simulink model "ANNpidSimulation"  (R2024b)
settings: Solver=ode45  StartTime=0.0  StopTime=5  FixedStep=1E-4  MaxStep=1E-4  RelTol=1E-3
undefined symbols (not defined in the file): initial_1, x, y, z
settings Model: Creator=b_ant  LastModifiedBy=b_ant
settings SolverCC: ZeroCrossAlgorithm=Adaptive
settings DebuggingCC: IgnoredZcDiagnostic=none  UnconnectedInputMsg=warning  UnconnectedOutputMsg=warning  UnconnectedLineMsg=warning
settings ModelReferenceCC: EnableRefExpFcnMdlSchedulingChecks=on
settings RTWCC: GPUComputeCapability=3.5  DLArmComputeVersion=19.05

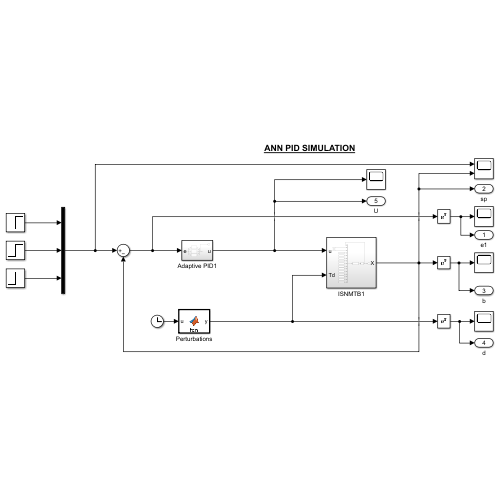
[thumbnail: Simulink's stored preview of the top-level diagram]
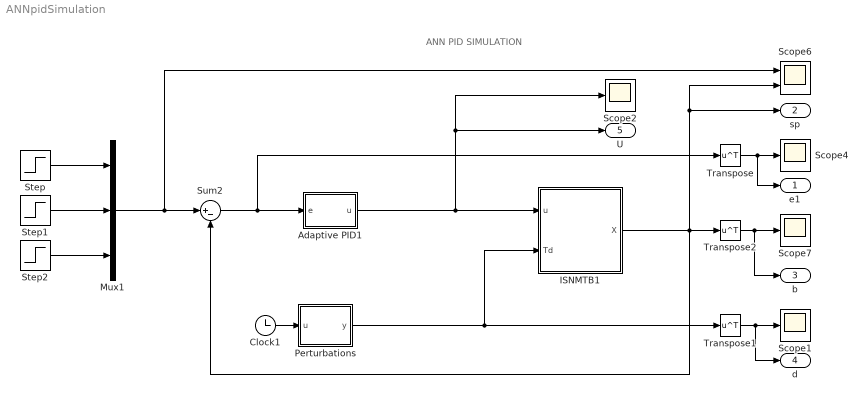
== system ANNpidSimulation ==
  note: ANN PID SIMULATION
  Adaptive PID1 : Subsystem
  Clock1 : Clock
      settings: Decimation=1000
  ISNMTB1 : Subsystem
  Mux1 : Mux  Inputs=3
  Perturbations : MATLAB Function  TreatAsAtomicUnit=on
  Scope{1..2,4,7} (4 alike) : Scope
  Scope6 : Scope  NumInputPorts=2
  Step : Step  Time=0.1  SampleTime=0
  Step1 : Step  Time=0.1  SampleTime=0
  Step2 : Step  Time=0.1  SampleTime=0
  Sum2 : Sum  Inputs=|+-
  Transpose : Math  Operator=transpose
  Transpose1 : Math  Operator=transpose
  Transpose2 : Math  Operator=transpose
  e1 : Outport
  sp : Outport  Port=2
  b : Outport  Port=3
  d : Outport  Port=4
  U : Outport  Port=5
  wires:
  Transpose1/1 -> Scope1/1, d/1
  ISNMTB1/1(X) -> sp/1, Scope6/2, Sum2/2, Transpose2/1
  Sum2/1 -> Transpose/1, Adaptive PID1/1(e)
  Step2/1 -> Mux1/3
  Transpose2/1 -> Scope7/1, b/1
  Step1/1 -> Mux1/2
  Clock1/1 -> Perturbations/1(u)
  Transpose/1 -> e1/1, Scope4/1
  Step/1 -> Mux1/1
  Mux1/1 -> Sum2/1, Scope6/1
  Perturbations/1(y) -> ISNMTB1/2(Td), Transpose1/1
  Adaptive PID1/1(u) -> U/1, Scope2/1, ISNMTB1/1(u)

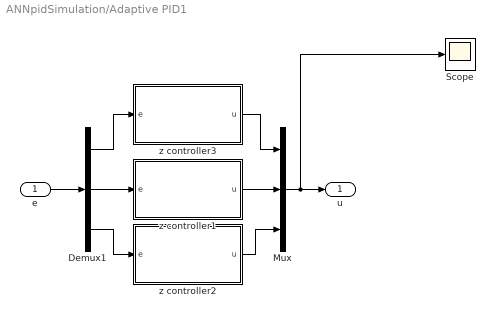
== system ANNpidSimulation/Adaptive PID1 ==
  e : Inport
  Demux1 : Demux  Outputs=3
  Mux : Mux  Inputs=3
  Scope : Scope
  z controller1 : Subsystem
  z controller2 : Subsystem
  z controller3 : Subsystem
  u : Outport
  wires:
  Demux1/2 -> z controller1/1(e)
  z controller3/1(u) -> Mux/1
  e/1 -> Demux1/1
  Demux1/1 -> z controller3/1(e)
  Mux/1 -> Scope/1, u/1
  Demux1/3 -> z controller2/1(e)
  z controller1/1(u) -> Mux/2
  z controller2/1(u) -> Mux/3

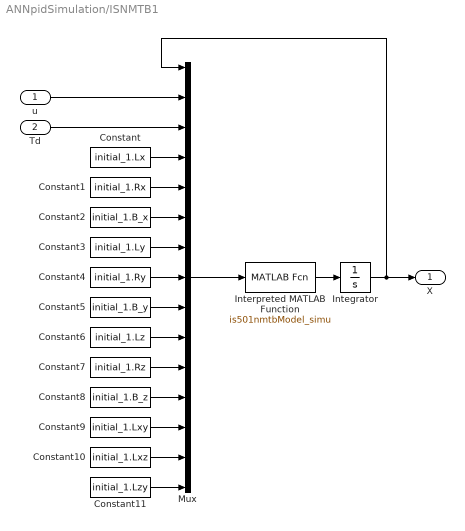
== system ANNpidSimulation/ISNMTB1 ==
  u : Inport
  Td : Inport  Port=2
  Constant : Constant  Value=initial_1.Lx
  Constant1 : Constant  Value=initial_1.Rx
  Constant10 : Constant  Value=initial_1.Lxz
  Constant11 : Constant  Value=initial_1.Lzy
  Constant2 : Constant  Value=initial_1.B_x
  Constant3 : Constant  Value=initial_1.Ly
  Constant4 : Constant  Value=initial_1.Ry
  Constant5 : Constant  Value=initial_1.B_y
  Constant6 : Constant  Value=initial_1.Lz
  Constant7 : Constant  Value=initial_1.Rz
  Constant8 : Constant  Value=initial_1.B_z
  Constant9 : Constant  Value=initial_1.Lxy
  Integrator : Integrator  InitialCondition=[3.249E4, -2.265E4, 3.655E4]
  Interpreted MATLAB Function : MATLABFcn  MATLABFcn=is501nmtbModel_simu
  Mux : Mux  Inputs=15
  X : Outport
  wires:
  Interpreted MATLAB Function/1 -> Integrator/1
  Integrator/1 -> X/1, Mux/1
  Mux/1 -> Interpreted MATLAB Function/1
  u/1 -> Mux/2
  Td/1 -> Mux/3
  Constant/1 -> Mux/4
  Constant1/1 -> Mux/5
  Constant2/1 -> Mux/6
  Constant3/1 -> Mux/7
  Constant4/1 -> Mux/8
  Constant5/1 -> Mux/9
  Constant6/1 -> Mux/10
  Constant7/1 -> Mux/11
  Constant8/1 -> Mux/12
  Constant9/1 -> Mux/13
  Constant10/1 -> Mux/14
  Constant11/1 -> Mux/15

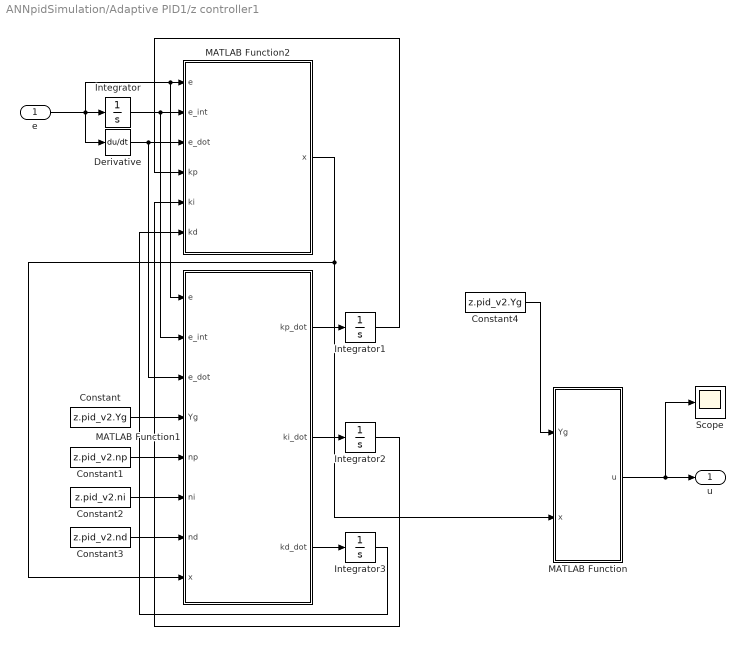
== system ANNpidSimulation/Adaptive PID1/z controller1 ==
  e : Inport
  Constant : Constant  Value=z.pid_v2.Yg
  Constant1 : Constant  Value=z.pid_v2.np
  Constant2 : Constant  Value=z.pid_v2.ni
  Constant3 : Constant  Value=z.pid_v2.nd
  Constant4 : Constant  Value=z.pid_v2.Yg
  Derivative : Derivative
  Integrator : Integrator
  Integrator1 : Integrator  InitialCondition=y.PID.Kp
  Integrator2 : Integrator  InitialCondition=y.PID.Ki
  Integrator3 : Integrator  InitialCondition=y.PID.Kd
  MATLAB Function : MATLAB Function  TreatAsAtomicUnit=on
  MATLAB Function1 : MATLAB Function  TreatAsAtomicUnit=on
  MATLAB Function2 : MATLAB Function  TreatAsAtomicUnit=on
  Scope : Scope
  u : Outport
  wires:
  e/1 -> Derivative/1, Integrator/1, MATLAB Function1/1(e), MATLAB Function2/1(e)
  Constant/1 -> MATLAB Function1/4(Yg)
  Constant1/1 -> MATLAB Function1/5(np)
  Constant2/1 -> MATLAB Function1/6(ni)
  Constant3/1 -> MATLAB Function1/7(nd)
  Constant4/1 -> MATLAB Function/1(Yg)
  MATLAB Function1/1(kp_dot) -> Integrator1/1
  MATLAB Function1/2(ki_dot) -> Integrator2/1
  MATLAB Function1/3(kd_dot) -> Integrator3/1
  Integrator/1 -> MATLAB Function1/2(e_int), MATLAB Function2/2(e_int)
  Derivative/1 -> MATLAB Function1/3(e_dot), MATLAB Function2/3(e_dot)
  MATLAB Function2/1(x) -> MATLAB Function/2(x), MATLAB Function1/8(x)
  Integrator1/1 -> MATLAB Function2/4(kp)
  Integrator2/1 -> MATLAB Function2/5(ki)
  Integrator3/1 -> MATLAB Function2/6(kd)
  MATLAB Function/1(u) -> Scope/1, u/1

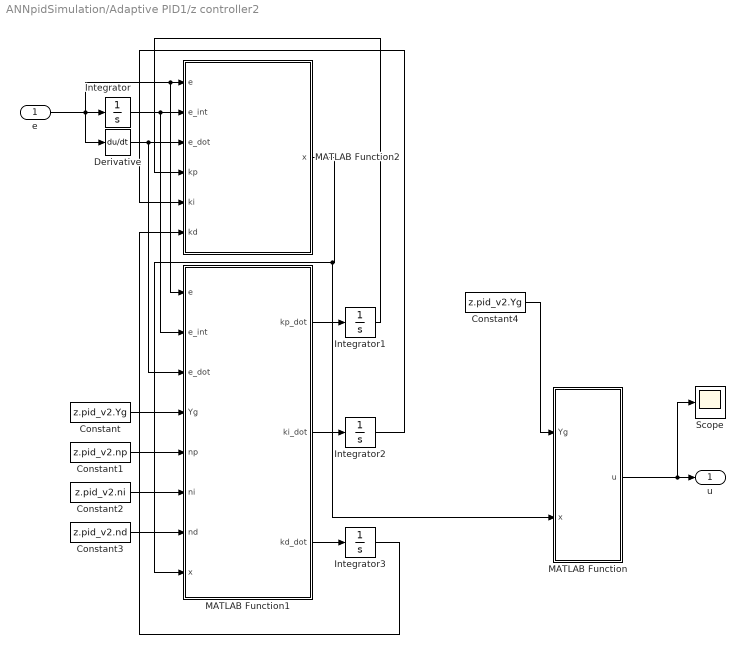
== system ANNpidSimulation/Adaptive PID1/z controller2 ==
  e : Inport
  Constant : Constant  Value=z.pid_v2.Yg
  Constant1 : Constant  Value=z.pid_v2.np
  Constant2 : Constant  Value=z.pid_v2.ni
  Constant3 : Constant  Value=z.pid_v2.nd
  Constant4 : Constant  Value=z.pid_v2.Yg
  Derivative : Derivative
  Integrator : Integrator
  Integrator1 : Integrator  InitialCondition=z.PID.Kp
  Integrator2 : Integrator  InitialCondition=z.PID.Ki
  Integrator3 : Integrator  InitialCondition=z.PID.Kd
  MATLAB Function : MATLAB Function  TreatAsAtomicUnit=on
  MATLAB Function1 : MATLAB Function  TreatAsAtomicUnit=on
  MATLAB Function2 : MATLAB Function  TreatAsAtomicUnit=on
  Scope : Scope
  u : Outport
  wires:
  e/1 -> Derivative/1, Integrator/1, MATLAB Function1/1(e), MATLAB Function2/1(e)
  Constant/1 -> MATLAB Function1/4(Yg)
  Constant1/1 -> MATLAB Function1/5(np)
  Constant2/1 -> MATLAB Function1/6(ni)
  Constant3/1 -> MATLAB Function1/7(nd)
  Constant4/1 -> MATLAB Function/1(Yg)
  MATLAB Function1/1(kp_dot) -> Integrator1/1
  MATLAB Function1/2(ki_dot) -> Integrator2/1
  MATLAB Function1/3(kd_dot) -> Integrator3/1
  Integrator/1 -> MATLAB Function1/2(e_int), MATLAB Function2/2(e_int)
  Derivative/1 -> MATLAB Function1/3(e_dot), MATLAB Function2/3(e_dot)
  MATLAB Function2/1(x) -> MATLAB Function/2(x), MATLAB Function1/8(x)
  Integrator1/1 -> MATLAB Function2/4(kp)
  Integrator2/1 -> MATLAB Function2/5(ki)
  Integrator3/1 -> MATLAB Function2/6(kd)
  MATLAB Function/1(u) -> Scope/1, u/1

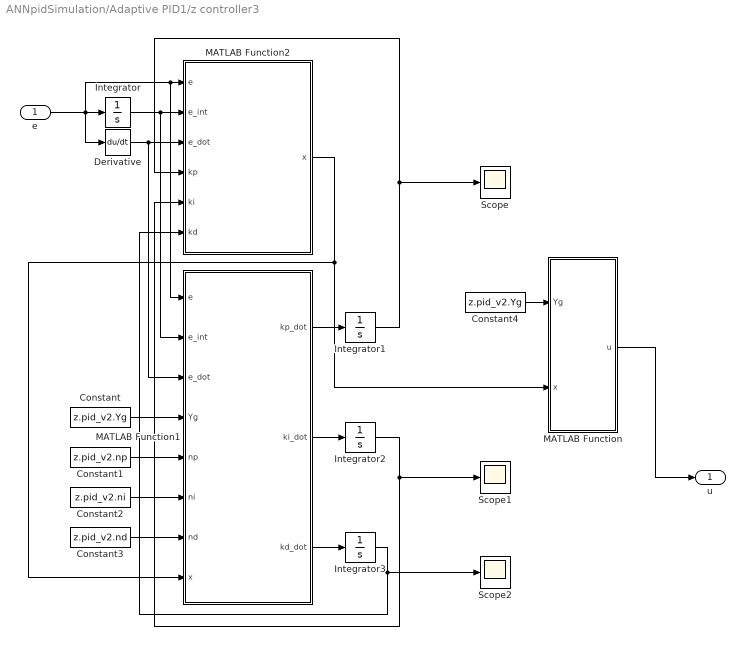
== system ANNpidSimulation/Adaptive PID1/z controller3 ==
  e : Inport
  Constant : Constant  Value=z.pid_v2.Yg
  Constant1 : Constant  Value=z.pid_v2.np
  Constant2 : Constant  Value=z.pid_v2.ni
  Constant3 : Constant  Value=z.pid_v2.nd
  Constant4 : Constant  Value=z.pid_v2.Yg
  Derivative : Derivative
  Integrator : Integrator
  Integrator1 : Integrator  InitialCondition=x.PID.Kp
  Integrator2 : Integrator  InitialCondition=x.PID.Ki
  Integrator3 : Integrator  InitialCondition=x.PID.Kd
  MATLAB Function : MATLAB Function  TreatAsAtomicUnit=on
  MATLAB Function1 : MATLAB Function  TreatAsAtomicUnit=on
  MATLAB Function2 : MATLAB Function  TreatAsAtomicUnit=on
  Scope : Scope
  Scope1 : Scope
  Scope2 : Scope
  u : Outport
  wires:
  e/1 -> Derivative/1, Integrator/1, MATLAB Function1/1(e), MATLAB Function2/1(e)
  Constant/1 -> MATLAB Function1/4(Yg)
  Constant1/1 -> MATLAB Function1/5(np)
  Constant2/1 -> MATLAB Function1/6(ni)
  Constant3/1 -> MATLAB Function1/7(nd)
  Constant4/1 -> MATLAB Function/1(Yg)
  MATLAB Function1/1(kp_dot) -> Integrator1/1
  MATLAB Function1/2(ki_dot) -> Integrator2/1
  MATLAB Function1/3(kd_dot) -> Integrator3/1
  Integrator/1 -> MATLAB Function1/2(e_int), MATLAB Function2/2(e_int)
  Derivative/1 -> MATLAB Function1/3(e_dot), MATLAB Function2/3(e_dot)
  MATLAB Function2/1(x) -> MATLAB Function/2(x), MATLAB Function1/8(x)
  Integrator1/1 -> Scope/1, MATLAB Function2/4(kp)
  Integrator2/1 -> MATLAB Function2/5(ki), Scope1/1
  Integrator3/1 -> Scope2/1, MATLAB Function2/6(kd)
  MATLAB Function/1(u) -> u/1

== matlab function ANNpidSimulation/Adaptive PID1/z controller2/MATLAB Function1 ==
  data: e input; kp_dot output; e_int input; e_dot input; Yg input; np input; ni input; nd input; ki_dot output; kd_dot output; x input
function [kp_dot,ki_dot,kd_dot] = neuronalPID(e,e_int,e_dot,Yg,np,ni,nd,x)
%e = entr(1);
%e_int = entr(2);
%e_dot = entr(3);
%x =  entr(4);
%Yg =  entr(5);
%np =  entr(6);
%ni =  entr(7);
%nd =  entr(8);
%kp_old
%ki_old
%kd_old 

kp_dot = np*e*e*sigmoid_dot(x, Yg);
ki_dot = ni*e*e_int*sigmoid_dot(x, Yg);
kd_dot = nd*e*e_dot*sigmoid_dot(x, Yg);
end

function f_dot = sigmoid_dot(x, Yg)
    f_dot = 4*exp(-x*Yg)/(1+exp(-x*Yg))^2;
end

== matlab function ANNpidSimulation/Adaptive PID1/z controller2/MATLAB Function2 ==
  data: e input; x output; e_int input; e_dot input; kp input; ki input; kd input
function x = myPidFun(e,e_int,e_dot,kp,ki,kd)
   x = kp*e+ki*e_int+kd*e_dot;
end

== matlab function ANNpidSimulation/Perturbations ==
  data: u input; y output
function y = fcn(u)
y= [2.522*sin(2*pi*4.788E-3*u)+3.249E04;
   -5.174*sin(2*pi*7.481E-3*u)-2.265E04;
    3.359*sin(2*pi*8.378E-3*u)+3.655E04];
end

== matlab function ANNpidSimulation/Adaptive PID1/z controller1/MATLAB Function ==
  data: Yg input; u output; x input
function u = fcn(Yg, x)
    u=sigmoid(x,Yg);
end

function f = sigmoid(x,Yg)
    f = 2/Yg * (1-exp(-x*Yg))/(1+exp(-x*Yg));
end

== matlab function ANNpidSimulation/Adaptive PID1/z controller1/MATLAB Function1 ==
  data: e input; kp_dot output; e_int input; e_dot input; Yg input; np input; ni input; nd input; ki_dot output; kd_dot output; x input
function [kp_dot,ki_dot,kd_dot] = neuronalPID(e,e_int,e_dot,Yg,np,ni,nd,x)
%e = entr(1);
%e_int = entr(2);
%e_dot = entr(3);
%x =  entr(4);
%Yg =  entr(5);
%np =  entr(6);
%ni =  entr(7);
%nd =  entr(8);
%kp_old
%ki_old
%kd_old 

kp_dot = np*e*e*sigmoid_dot(x, Yg);
ki_dot = ni*e*e_int*sigmoid_dot(x, Yg);
kd_dot = nd*e*e_dot*sigmoid_dot(x, Yg);
end

function f_dot = sigmoid_dot(x, Yg)
    f_dot = 4*exp(-x*Yg)/(1+exp(-x*Yg))^2;
end

== matlab function ANNpidSimulation/Adaptive PID1/z controller3/MATLAB Function ==
  data: Yg input; u output; x input
function u = fcn(Yg, x)
    u=sigmoid(x,Yg);
end

function f = sigmoid(x,Yg)
    f = 2/Yg * (1-exp(-x*Yg))/(1+exp(-x*Yg));
end

== matlab function ANNpidSimulation/Adaptive PID1/z controller3/MATLAB Function1 ==
  data: e input; kp_dot output; e_int input; e_dot input; Yg input; np input; ni input; nd input; ki_dot output; kd_dot output; x input
function [kp_dot,ki_dot,kd_dot] = neuronalPID(e,e_int,e_dot,Yg,np,ni,nd,x)
%e = entr(1);
%e_int = entr(2);
%e_dot = entr(3);
%x =  entr(4);
%Yg =  entr(5);
%np =  entr(6);
%ni =  entr(7);
%nd =  entr(8);
%kp_old
%ki_old
%kd_old 

kp_dot = np*e*e*sigmoid_dot(x, Yg);
ki_dot = ni*e*e_int*sigmoid_dot(x, Yg);
kd_dot = nd*e*e_dot*sigmoid_dot(x, Yg);
end

function f_dot = sigmoid_dot(x, Yg)
    f_dot = 4*exp(-x*Yg)/(1+exp(-x*Yg))^2;
end

== matlab function ANNpidSimulation/Adaptive PID1/z controller1/MATLAB Function2 ==
  data: e input; x output; e_int input; e_dot input; kp input; ki input; kd input
function x = myPidFun(e,e_int,e_dot,kp,ki,kd)
   x = kp*e+ki*e_int+kd*e_dot;
end

== matlab function ANNpidSimulation/Adaptive PID1/z controller2/MATLAB Function ==
  data: Yg input; u output; x input
function u = fcn(Yg, x)
    u=sigmoid(x,Yg);
end

function f = sigmoid(x,Yg)
    f = 2/Yg * (1-exp(-x*Yg))/(1+exp(-x*Yg));
end

== matlab function ANNpidSimulation/Adaptive PID1/z controller3/MATLAB Function2 ==
  data: e input; x output; e_int input; e_dot input; kp input; ki input; kd input
function x = myPidFun(e,e_int,e_dot,kp,ki,kd)
   x = kp*e+ki*e_int+kd*e_dot;
end
